simulink library "mech_stewart_controllers"  (Simulink 7.1)
values from neighbouring files (symbols this model uses):
  Ak = [-1697.70247289 -84.8146549606 -57.1718135112 270.473316945 -57.171813483 12.9581182618 -530032.227354 -51423.5874655 -37197.2166541 203871.174251 -37141.5821622 18540.2571033 ... (324 elements, 18x18)]    [mech_stewart_control_Hinf.mat]
  Bk = [1697.70247289 84.8146549606 57.1718135112 -270.473316945 57.171813483 -12.9581182618 444258.815048 42487.6011968 30423.7625952 -164792.340046 30370.0437282 -14348.6043858 ... (216 elements, 18x12)]    [mech_stewart_control_Hinf.mat]
  Ck = [-1.00011609263 5.97678206219e-05 3.18868867016e-05 -2.514712894e-05 7.64338569004e-06 -9.44720298065e-06 -9.44724487133e-06 7.6433999019e-06 -2.51471714827e-05 3.18868934787e-05 5.97678371914e-05 -1.00011609263 ... (108 elements, 6x18)]    [mech_stewart_control_Hinf.mat]
  Dk = [0 0 0 0 0 0 0 0 0 0 0 0 ... (72 elements, 6x12)]    [mech_stewart_control_Hinf.mat]
  force_act_max = 3e5    (= 300000)    [mech_stewart_studies_setup.m]
  initCondI = (upper_leg_mass+lower_leg_mass+(top_mass*1.3/6))*9.81/Ki    [mech_stewart_studies_setup.m]
  Kd = 4.5e4    (= 45000)    [mech_stewart_studies_setup.m]    (also in mech_stewartplatform_dat.m)
  Ki = 1e4    (= 10000)    [mech_stewart_studies_setup.m]    (also in mech_stewartplatform_dat.m)
  Kp = 2e6    (= 2000000)    [mech_stewart_studies_setup.m]    (also in mech_stewartplatform_dat.m)
libraries: mech_stewart_controllers x1
settings Model: Creator=jwendlan  LastModifiedBy=batserve  ExtModeAutoUpdateStatusClock=off

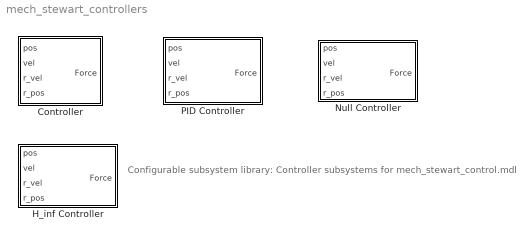
== system mech_stewart_controllers ==
  note: Configurable subsystem library:
      | Controller subsystems for
      | mech_stewart_control.mdl
  "Controller " : Subsystem  BlockChoice=Null Controller
      settings: TemplateBlock=self  MemberBlocks=H_inf Controller,Null Controller,PID Controller
  H_inf Controller : Subsystem
  Null Controller : Subsystem
  PID Controller : Subsystem

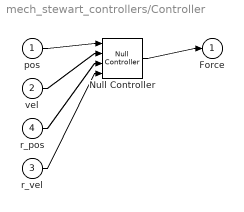
== system mech_stewart_controllers/Controller  ==
  pos : Inport  OutDataType=sfix(16)  OutScaling=2^0
  vel : Inport  Port=2  OutDataType=sfix(16)  OutScaling=2^0
  r_vel : Inport  Port=3  OutDataType=sfix(16)  OutScaling=2^0
  r_pos : Inport  Port=4  OutDataType=sfix(16)  OutScaling=2^0
  Null Controller : mech_stewart_controllers/Null Controller  SystemSampleTime=-1
  Force : Outport  OutDataType=sfix(16)  OutScaling=2^0
  wires:
  pos/1 -> Null Controller/1
  vel/1 -> Null Controller/2
  r_pos/1 -> Null Controller/3
  r_vel/1 -> Null Controller/4
  Null Controller/1 -> Force/1

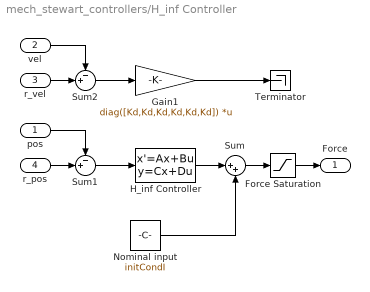
== system mech_stewart_controllers/H_inf Controller ==
  pos : Inport  OutDataType=sfix(16)  OutScaling=2^0
  vel : Inport  Port=2  OutDataType=sfix(16)  OutScaling=2^0
  r_vel : Inport  Port=3  OutDataType=sfix(16)  OutScaling=2^0
  r_pos : Inport  Port=4  OutDataType=sfix(16)  OutScaling=2^0
  Force Saturation : Saturate  UpperLimit=force_act_max  LowerLimit=-force_act_max  LinearizeAsGain=off  ZeroCross=off
  Gain1 : Gain  Gain=diag([Kd,Kd,Kd,Kd,Kd,Kd])  Multiplication=Matrix(K*u)  ParameterDataType=sfix(16)  ParameterScaling=2^0  OutDataType=sfix(16)  OutScaling=2^0  SaturateOnIntegerOverflow=on  OutDataTypeStr=Inherit: Same as input  ParamDataTypeStr=Inherit: Same as input
  H_inf Controller : StateSpace  A=Ak  B=Bk  C=Ck  D=Dk
  Nominal input : Constant  Value=initCondI  OutDataType=sfix(16)  OutScaling=2^0
  Sum : Sum  Inputs=|++  OutDataType=sfix(16)  OutScaling=2^0
  Sum1 : Sum  Inputs=-+|  OutDataType=sfix(16)  OutScaling=2^0  SaturateOnIntegerOverflow=on  InputSameDT=on  OutDataTypeStr=Inherit: Same as first input
  Sum2 : Sum  Inputs=-+|  OutDataType=sfix(16)  OutScaling=2^0  SaturateOnIntegerOverflow=on  InputSameDT=on  OutDataTypeStr=Inherit: Same as first input
  Terminator : Terminator
  Force : Outport  OutDataType=sfix(16)  OutScaling=2^0
  wires:
  pos/1 -> Sum1/1
  r_pos/1 -> Sum1/2
  Sum1/1 -> H_inf Controller/1
  r_vel/1 -> Sum2/2
  vel/1 -> Sum2/1
  Sum2/1 -> Gain1/1
  Nominal input/1 -> Sum/2
  Sum/1 -> Force Saturation/1
  Force Saturation/1 -> Force/1
  Gain1/1 -> Terminator/1
  H_inf Controller/1 -> Sum/1

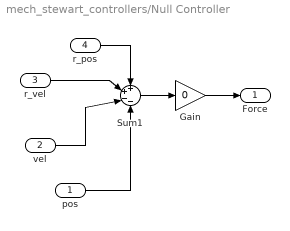
== system mech_stewart_controllers/Null Controller ==
  pos : Inport  OutDataType=sfix(16)  OutScaling=2^0
  vel : Inport  Port=2  OutDataType=sfix(16)  OutScaling=2^0
  r_vel : Inport  Port=3  OutDataType=sfix(16)  OutScaling=2^0
  r_pos : Inport  Port=4  OutDataType=sfix(16)  OutScaling=2^0
  Gain : Gain  Gain=0  ParameterDataType=sfix(16)  ParameterScaling=2^0  OutDataType=sfix(16)  OutScaling=2^0
  Sum1 : Sum  Inputs=++--  OutDataType=sfix(16)  OutScaling=2^0  SaturateOnIntegerOverflow=on  InputSameDT=on  OutDataTypeStr=Inherit: Same as first input
  Force : Outport  OutDataType=sfix(16)  OutScaling=2^0
  wires:
  Gain/1 -> Force/1
  Sum1/1 -> Gain/1
  pos/1 -> Sum1/4
  vel/1 -> Sum1/3
  r_pos/1 -> Sum1/1
  r_vel/1 -> Sum1/2

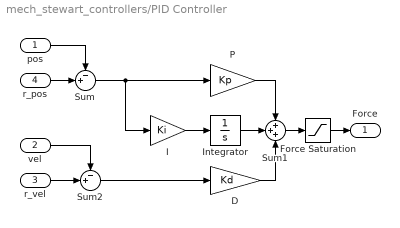
== system mech_stewart_controllers/PID Controller ==
  pos : Inport  OutDataType=sfix(16)  OutScaling=2^0
  vel : Inport  Port=2  OutDataType=sfix(16)  OutScaling=2^0
  r_vel : Inport  Port=3  OutDataType=sfix(16)  OutScaling=2^0
  r_pos : Inport  Port=4  OutDataType=sfix(16)  OutScaling=2^0
  "   I" : Gain  Gain=Ki  ParameterDataType=sfix(16)  ParameterScaling=2^0  OutDataType=sfix(16)  OutScaling=2^0  SaturateOnIntegerOverflow=on  OutDataTypeStr=Inherit: Same as input  ParamDataTypeStr=Inherit: Same as input
  D : Gain  Gain=Kd  ParameterDataType=sfix(16)  ParameterScaling=2^0  OutDataType=sfix(16)  OutScaling=2^0  SaturateOnIntegerOverflow=on  OutDataTypeStr=Inherit: Same as input  ParamDataTypeStr=Inherit: Same as input
  Force Saturation : Saturate  UpperLimit=force_act_max  LowerLimit=-force_act_max  LinearizeAsGain=off  ZeroCross=off
  Integrator : Integrator  InitialCondition=initCondI  ZeroCross=off
  P : Gain  Gain=Kp  ParameterDataType=sfix(16)  ParameterScaling=2^0  OutDataType=sfix(16)  OutScaling=2^0  SaturateOnIntegerOverflow=on  OutDataTypeStr=Inherit: Same as input  ParamDataTypeStr=Inherit: Same as input
  Sum : Sum  Inputs=-+|  OutDataType=sfix(16)  OutScaling=2^0  SaturateOnIntegerOverflow=on  InputSameDT=on  OutDataTypeStr=Inherit: Same as first input
  Sum1 : Sum  Inputs=+++  OutDataType=sfix(16)  OutScaling=2^0  SaturateOnIntegerOverflow=on  InputSameDT=on  OutDataTypeStr=Inherit: Same as first input
  Sum2 : Sum  Inputs=-+|  OutDataType=sfix(16)  OutScaling=2^0  SaturateOnIntegerOverflow=on  InputSameDT=on  OutDataTypeStr=Inherit: Same as first input
  Force : Outport  OutDataType=sfix(16)  OutScaling=2^0
  wires:
  r_pos/1 -> Sum/2
  pos/1 -> Sum/1
  D/1 -> Sum1/3
  P/1 -> Sum1/1
  Sum/1 -> P/1, "   I"/1
  vel/1 -> Sum2/1
  r_vel/1 -> Sum2/2
  Sum2/1 -> D/1
  Sum1/1 -> Force Saturation/1
  Force Saturation/1 -> Force/1
  "   I"/1 -> Integrator/1
  Integrator/1 -> Sum1/2
